simulink model "gm_sampleModel1581_2_sub"  (R2023a)
settings: Solver=VariableStepAuto  StartTime=0.0  StopTime=10.0  RelTol=1e-3
libraries: simulink x3, hdlsllib x1
settings Model: Creator=user1  LastModifiedBy=user1
settings OptimizationCC: BlockReduction=off  ConditionallyExecuteInputs=off
settings DebuggingCC: InheritedTsInSrcMsg=none

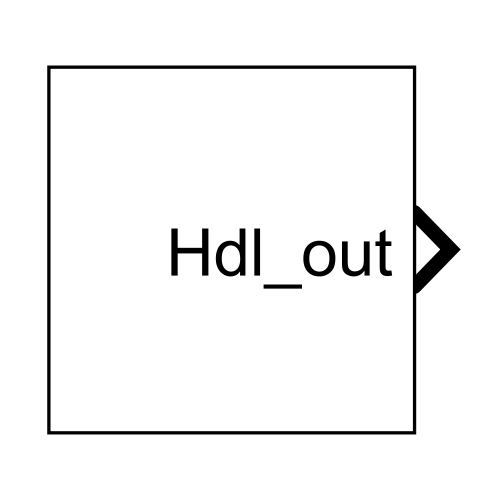
[thumbnail: Simulink's stored preview of the top-level diagram]
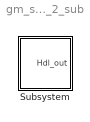
== system gm_sampleModel1581_2_sub ==
  Subsystem : Subsystem

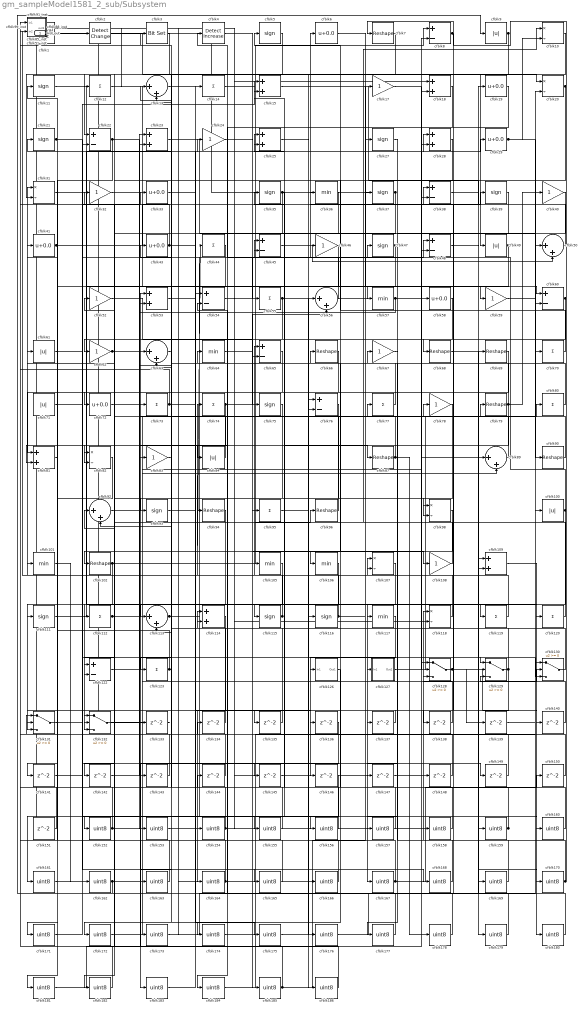
== system gm_sampleModel1581_2_sub/Subsystem ==
  cfblk1 : hdlsllib/Logic and Bit Operations/Interval Test  IntervalClosedRight=on  uplimit=0.5  IntervalClosedLeft=on  lowlimit=-0.5  OutDataTypeStr=uint8
  cfblk{10,20,31,82,98,107,118} (7 alike) : Product  Inputs=*/  OutDataTypeStr=uint8  RndMeth=Zero  SaturateOnIntegerOverflow=on
  cfblk{9,49,61,71,84,100} (6 alike) : Abs  OutDataTypeStr=uint8  SaturateOnIntegerOverflow=off
  cfblk{36,57,64,101,105..106,117} (7 alike) : MinMax  OutDataTypeStr=uint8
  cfblk{7,66,68..69,79,87,90,94,96,102} (10 alike) : Reshape
  cfblk{17,24,32,40,46,52,59,62,67,78,83,108} (12 alike) : Gain  OutDataTypeStr=uint8
  cfblk{15,18,23,25,28,53,81,109,114} (9 alike) : Sum  OutDataTypeStr=uint8
  cfblk{5,11,21,27,35,37,39,47,75,93,111,115..116} (13 alike) : Signum
  cfblk{12,14,44,55,70,73..74,77,80,95,112,119..120,123} (14 alike) : Sum  Inputs=+  OutDataTypeStr=uint8
  cfblk{13,50,56,63,89,92,113} (7 alike) : Sum  Inputs=|++  OutDataTypeStr=uint8
  cfblk{8,22,38,45,48,54,60,65,76,122} (10 alike) : Sum  Inputs=+-  OutDataTypeStr=uint8
  cfblk126 : Subsystem
  cfblk127 : Subsystem
  cfblk{128..132} (5 alike) : Switch  OutDataTypeStr=uint8  SaturateOnIntegerOverflow=off  InputSameDT=off
  cfblk{133..151} (19 alike) : Delay  SampleTime=1
  cfblk{152..186} (35 alike) : DataTypeConversion  OutDataTypeStr=uint8  SaturateOnIntegerOverflow=off  RndMeth=Floor
  cfblk16_inst : Subsystem
  cfblk{6,19,29,33,41,43,58,72} (8 alike) : Bias  Bias=0.0  SaturateOnIntegerOverflow=off
  cfblk2 : simulink/Logic and Bit Operations/Detect Change  vinit=0  OutDataTypeStr=uint8
      settings: LibrarySourceBlock=|
      | hdlsllib/Logic and Bit
      | Operations/Detect
      | Change
  cfblk26_inst : Subsystem
  cfblk3 : simulink/Logic and Bit Operations/Bit Set  iBit=0
      settings: LibrarySourceBlock=|
      | hdlsllib/Logic and Bit
      | Operations/Bit Set
  cfblk4 : simulink/Logic and Bit Operations/Detect Increase  vinit=0.0  OutDataTypeStr=uint8
      settings: LibrarySourceBlock=|
      | hdlsllib/Logic and Bit
      | Operations/Detect
      | Increase
  cfblk51_inst : Subsystem
  cfblk85_inst : Subsystem
  cfblk88_inst : Subsystem
  cfblk91_inst : Subsystem
  cfblk99_inst : Subsystem
  Hdl_out : Outport  OutDataTypeStr=uint8  SampleTime=1
  wires:
  cfblk1/1 -> cfblk2/1
  cfblk10/1 -> cfblk49/1
  cfblk100/1 -> cfblk47/1, cfblk132/3
  cfblk101/1 -> cfblk162/1
  cfblk102/1 -> cfblk96/1, cfblk8/1, cfblk122/2, cfblk44/1
  cfblk105/1 -> cfblk132/2
  cfblk106/1 -> cfblk131/3
  cfblk107/1 -> cfblk167/1
  cfblk108/1 -> cfblk10/1
  cfblk109/1 -> cfblk180/1
  cfblk11/1 -> cfblk120/1
  cfblk111/1 -> cfblk29/1
  cfblk112/1 -> cfblk89/2, cfblk117/1
  cfblk113/1 -> cfblk6/1, cfblk156/1
  cfblk114/1 -> cfblk164/1
  cfblk115/1 -> cfblk65/1, cfblk53/1, cfblk31/1
  cfblk116/1 -> cfblk119/1, cfblk73/1
  cfblk117/1 -> cfblk146/1
  cfblk118/1 -> cfblk74/1
  cfblk119/1 -> cfblk16_inst/2(in2)
  cfblk12/1 -> cfblk75/1
  cfblk120/1 -> cfblk61/1
  cfblk122/1 -> cfblk126/1(In1)
  cfblk123/1 -> cfblk63/1, cfblk11/1
  cfblk126/1(Out1) -> cfblk172/1
  cfblk127/1(Out1) -> cfblk79/1
  cfblk128/1 -> cfblk140/1, cfblk139/1
  cfblk129/1 -> cfblk92/2, cfblk63/2, cfblk135/1, cfblk77/1
  cfblk13/1 -> cfblk154/1
  cfblk130/1 -> cfblk45/1
  cfblk131/1 -> cfblk33/1
  cfblk132/1 -> cfblk37/1
  cfblk133/1 -> cfblk1/1
  cfblk134/1 -> cfblk91_inst/2(in2)
  cfblk135/1 -> cfblk54/2
  cfblk136/1 -> cfblk183/1
  cfblk137/1 -> cfblk131/2
  cfblk138/1 -> cfblk118/1
  cfblk139/1 -> cfblk20/2
  cfblk14/1 -> cfblk20/1
  cfblk140/1 -> cfblk129/3
  cfblk141/1 -> cfblk22/2
  cfblk142/1 -> cfblk23/2
  cfblk143/1 -> cfblk131/1
  cfblk144/1 -> cfblk16_inst/1(in1)
  cfblk145/1 -> cfblk56/1
  cfblk146/1 -> cfblk161/1
  cfblk147/1 -> cfblk18/2
  cfblk148/1 -> cfblk25/1
  cfblk149/1 -> cfblk129/2
  cfblk15/1 -> cfblk159/1
  cfblk150/1 -> cfblk85_inst/1(in1)
  cfblk151/1 -> cfblk51_inst/2(in2)
  cfblk152/1 -> cfblk27/1, cfblk26_inst/2(in2)
  cfblk153/1 -> cfblk78/1
  cfblk154/1 -> cfblk100/1, cfblk144/1
  cfblk155/1 -> cfblk13/1
  cfblk156/1 -> cfblk13/2
  cfblk157/1 -> cfblk66/1
  cfblk158/1 -> cfblk67/1
  cfblk159/1 -> cfblk41/1, cfblk83/1
  cfblk16_inst/1(out1) -> cfblk18/1
  cfblk160/1 -> cfblk15/1
  cfblk161/1 -> cfblk15/2
  cfblk162/1 -> cfblk9/1, cfblk130/2, cfblk105/1
  cfblk163/1 -> cfblk101/1
  cfblk164/1 -> cfblk88_inst/2(in2), cfblk88_inst/1(in1), cfblk130/1, cfblk109/1
  cfblk165/1 -> cfblk114/1
  cfblk166/1 -> cfblk114/2
  cfblk167/1 -> cfblk92/1, cfblk150/1
  cfblk168/1 -> cfblk107/1
  cfblk169/1 -> cfblk107/2
  cfblk17/1 -> cfblk89/1
  cfblk170/1 -> cfblk7/1, cfblk128/3
  cfblk171/1 -> cfblk48/1
  cfblk172/1 -> cfblk48/2
  cfblk173/1 -> cfblk50/1
  cfblk174/1 -> cfblk76/1
  cfblk175/1 -> cfblk76/2
  cfblk176/1 -> cfblk69/1
  cfblk177/1 -> cfblk99_inst/1(in1)
  cfblk178/1 -> cfblk99_inst/2(in2)
  cfblk179/1 -> cfblk134/1
  cfblk18/1 -> cfblk184/1
  cfblk180/1 -> cfblk38/1
  cfblk181/1 -> cfblk38/2
  cfblk182/1 -> cfblk91_inst/1(in1)
  cfblk183/1 -> cfblk28/1
  cfblk184/1 -> cfblk28/2
  cfblk185/1 -> cfblk51_inst/1(in1), cfblk17/1, cfblk133/1
  cfblk186/1 -> cfblk52/1
  cfblk19/1 -> cfblk94/1
  cfblk2/1 -> cfblk116/1
  cfblk20/1 -> cfblk98/2, cfblk98/1, cfblk106/1
  cfblk21/1 -> cfblk165/1, cfblk149/1
  cfblk22/1 -> cfblk130/3, cfblk111/1
  cfblk23/1 -> cfblk90/1
  cfblk24/1 -> cfblk55/1
  cfblk25/1 -> cfblk186/1
  cfblk26_inst/1(out1) -> cfblk148/1
  cfblk27/1 -> cfblk147/1
  cfblk28/1 -> cfblk182/1
  cfblk29/1 -> cfblk60/2, cfblk10/2
  cfblk3/1 -> cfblk31/2
  cfblk31/1 -> cfblk128/1
  cfblk32/1 -> cfblk57/1
  cfblk33/1 -> cfblk54/1
  cfblk35/1 -> cfblk155/1, cfblk62/1
  cfblk36/1 -> cfblk82/2
  cfblk37/1 -> cfblk84/1, Hdl_out/1
  cfblk38/1 -> cfblk179/1
  cfblk39/1 -> cfblk137/1
  cfblk4/1 -> cfblk95/1
  cfblk40/1 -> cfblk109/2
  cfblk41/1 -> cfblk60/1, cfblk19/1
  cfblk43/1 -> cfblk85_inst/2(in2), cfblk136/1
  cfblk44/1 -> cfblk171/1
  cfblk45/1 -> cfblk50/2
  cfblk46/1 -> cfblk72/1
  cfblk47/1 -> cfblk45/2, cfblk145/1
  cfblk48/1 -> cfblk170/1
  cfblk49/1 -> cfblk177/1, cfblk174/1
  cfblk5/1 -> cfblk163/1
  cfblk50/1 -> cfblk36/1
  cfblk51_inst/1(out1) -> cfblk166/1, cfblk118/2
  cfblk52/1 -> cfblk185/1
  cfblk53/1 -> cfblk39/1
  cfblk54/1 -> cfblk46/1
  cfblk55/1 -> cfblk65/2, cfblk113/1
  cfblk56/1 -> cfblk4/1
  cfblk57/1 -> cfblk8/2, cfblk53/2
  cfblk58/1 -> cfblk102/1
  cfblk59/1 -> cfblk70/1
  cfblk6/1 -> cfblk59/1
  cfblk60/1 -> cfblk128/2, cfblk142/1
  cfblk61/1 -> cfblk127/1(In1)
  cfblk62/1 -> cfblk153/1, cfblk24/1
  cfblk63/1 -> cfblk93/1
  cfblk64/1 -> cfblk108/1
  cfblk65/1 -> cfblk112/1
  cfblk66/1 -> cfblk82/1
  cfblk67/1 -> cfblk157/1
  cfblk68/1 -> cfblk169/1
  cfblk69/1 -> cfblk81/1
  cfblk7/1 -> cfblk132/1
  cfblk70/1 -> cfblk5/1
  cfblk71/1 -> cfblk160/1
  cfblk72/1 -> cfblk87/1
  cfblk73/1 -> cfblk26_inst/1(in1), cfblk168/1
  cfblk74/1 -> cfblk81/2, cfblk56/2
  cfblk75/1 -> cfblk143/1
  cfblk76/1 -> cfblk173/1
  cfblk77/1 -> cfblk43/1
  cfblk78/1 -> cfblk152/1
  cfblk79/1 -> cfblk35/1, cfblk115/1, cfblk40/1
  cfblk8/1 -> cfblk68/1, cfblk138/1
  cfblk80/1 -> cfblk21/1
  cfblk81/1 -> cfblk181/1
  cfblk82/1 -> cfblk141/1
  cfblk83/1 -> cfblk113/2
  cfblk84/1 -> cfblk3/1
  cfblk85_inst/1(out1) -> cfblk58/1, cfblk158/1, cfblk151/1
  cfblk87/1 -> cfblk23/1, cfblk178/1
  cfblk88_inst/1(out1) -> cfblk71/1
  cfblk89/1 -> cfblk64/1
  cfblk9/1 -> cfblk22/1, cfblk12/1
  cfblk90/1 -> cfblk25/2
  cfblk91_inst/1(out1) -> cfblk14/1
  cfblk92/1 -> cfblk80/1
  cfblk93/1 -> cfblk175/1
  cfblk94/1 -> cfblk123/1
  cfblk95/1 -> cfblk129/1
  cfblk96/1 -> cfblk32/1
  cfblk98/1 -> cfblk122/1
  cfblk99_inst/1(out1) -> cfblk176/1

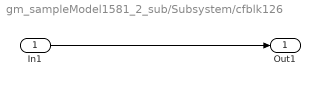
== system gm_sampleModel1581_2_sub/Subsystem/cfblk126 ==
  In1 : Inport  OutDataTypeStr=uint8  PortDimensions=1  SampleTime=1
  Out1 : Outport  SampleTime=1
  wires:
  In1/1 -> Out1/1

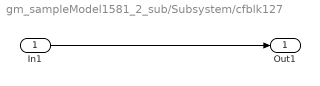
== system gm_sampleModel1581_2_sub/Subsystem/cfblk127 ==
  In1 : Inport  OutDataTypeStr=uint8  PortDimensions=1  SampleTime=1
  Out1 : Outport  SampleTime=1
  wires:
  In1/1 -> Out1/1

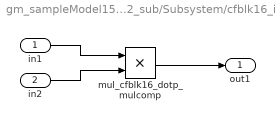
== system gm_sampleModel1581_2_sub/Subsystem/cfblk16_inst ==
  in1 : Inport  OutDataTypeStr=uint8  SampleTime=1
  in2 : Inport  Port=2  OutDataTypeStr=uint8  SampleTime=1
  mul_cfblk16_dotp_mulcomp : Product  Inputs=**  OutDataTypeStr=uint8  SampleTime=1
  out1 : Outport  OutDataTypeStr=uint8  SampleTime=1
  wires:
  in1/1 -> mul_cfblk16_dotp_mulcomp/1
  in2/1 -> mul_cfblk16_dotp_mulcomp/2
  mul_cfblk16_dotp_mulcomp/1 -> out1/1

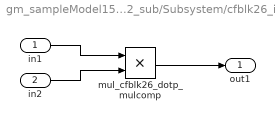
== system gm_sampleModel1581_2_sub/Subsystem/cfblk26_inst ==
  in1 : Inport  OutDataTypeStr=uint8  SampleTime=1
  in2 : Inport  Port=2  OutDataTypeStr=uint8  SampleTime=1
  mul_cfblk26_dotp_mulcomp : Product  Inputs=**  OutDataTypeStr=uint8  SampleTime=1
  out1 : Outport  OutDataTypeStr=uint8  SampleTime=1
  wires:
  in1/1 -> mul_cfblk26_dotp_mulcomp/1
  in2/1 -> mul_cfblk26_dotp_mulcomp/2
  mul_cfblk26_dotp_mulcomp/1 -> out1/1

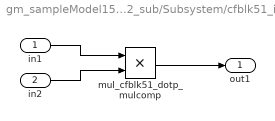
== system gm_sampleModel1581_2_sub/Subsystem/cfblk51_inst ==
  in1 : Inport  OutDataTypeStr=uint8  SampleTime=1
  in2 : Inport  Port=2  OutDataTypeStr=uint8  SampleTime=1
  mul_cfblk51_dotp_mulcomp : Product  Inputs=**  OutDataTypeStr=uint8  SampleTime=1
  out1 : Outport  OutDataTypeStr=uint8  SampleTime=1
  wires:
  in1/1 -> mul_cfblk51_dotp_mulcomp/1
  in2/1 -> mul_cfblk51_dotp_mulcomp/2
  mul_cfblk51_dotp_mulcomp/1 -> out1/1

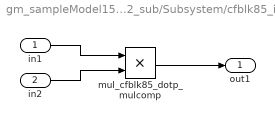
== system gm_sampleModel1581_2_sub/Subsystem/cfblk85_inst ==
  in1 : Inport  OutDataTypeStr=uint8  SampleTime=1
  in2 : Inport  Port=2  OutDataTypeStr=uint8  SampleTime=1
  mul_cfblk85_dotp_mulcomp : Product  Inputs=**  OutDataTypeStr=uint8  SampleTime=1
  out1 : Outport  OutDataTypeStr=uint8  SampleTime=1
  wires:
  in1/1 -> mul_cfblk85_dotp_mulcomp/1
  in2/1 -> mul_cfblk85_dotp_mulcomp/2
  mul_cfblk85_dotp_mulcomp/1 -> out1/1

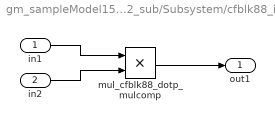
== system gm_sampleModel1581_2_sub/Subsystem/cfblk88_inst ==
  in1 : Inport  OutDataTypeStr=uint8  SampleTime=1
  in2 : Inport  Port=2  OutDataTypeStr=uint8  SampleTime=1
  mul_cfblk88_dotp_mulcomp : Product  Inputs=**  OutDataTypeStr=uint8  SampleTime=1
  out1 : Outport  OutDataTypeStr=uint8  SampleTime=1
  wires:
  in1/1 -> mul_cfblk88_dotp_mulcomp/1
  in2/1 -> mul_cfblk88_dotp_mulcomp/2
  mul_cfblk88_dotp_mulcomp/1 -> out1/1

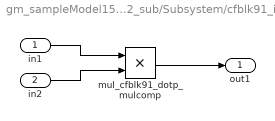
== system gm_sampleModel1581_2_sub/Subsystem/cfblk91_inst ==
  in1 : Inport  OutDataTypeStr=uint8  SampleTime=1
  in2 : Inport  Port=2  OutDataTypeStr=uint8  SampleTime=1
  mul_cfblk91_dotp_mulcomp : Product  Inputs=**  OutDataTypeStr=uint8  SampleTime=1
  out1 : Outport  OutDataTypeStr=uint8  SampleTime=1
  wires:
  in1/1 -> mul_cfblk91_dotp_mulcomp/1
  in2/1 -> mul_cfblk91_dotp_mulcomp/2
  mul_cfblk91_dotp_mulcomp/1 -> out1/1

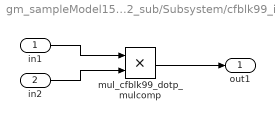
== system gm_sampleModel1581_2_sub/Subsystem/cfblk99_inst ==
  in1 : Inport  OutDataTypeStr=uint8  SampleTime=1
  in2 : Inport  Port=2  OutDataTypeStr=uint8  SampleTime=1
  mul_cfblk99_dotp_mulcomp : Product  Inputs=**  OutDataTypeStr=uint8  SampleTime=1
  out1 : Outport  OutDataTypeStr=uint8  SampleTime=1
  wires:
  in1/1 -> mul_cfblk99_dotp_mulcomp/1
  in2/1 -> mul_cfblk99_dotp_mulcomp/2
  mul_cfblk99_dotp_mulcomp/1 -> out1/1
